simulink model "pv_trial"  (R2013a)
settings: Solver=ode4  StartTime=0.0  StopTime=0.2  FixedStep=1e-5  MaxStep=1e-5  RelTol=1e-3
values from neighbouring files (symbols this model uses):
  delta = atan(Idpv*Xs/(Vs-Iqpv*Xs))*180/pi    [rpg_simulation_base.m]
  fs = 50    [rpg_loss_calculation.m]    (also in rpg_simulation_base.m)
  fsw = 5e3    (= 5000)    [calculate_loss.m]    (also in rpg_loss_calculation.m; rpg_simulation_base.m = 2000)
  Ls = 1e-3    (= 0.001)    [rpg_simulation_base.m]
  ma = Vc_mag*sqrt(2)/Vdc    [rpg_simulation_base.m]
  Vdc = 750    [calculate_loss.m]    (also in rpg_loss_calculation.m; rpg_simulation_base.m)
  Vs = 400    [rpg_simulation_base.m]
libraries: powerlib x11, powerlib_extras x6, powerlib_meascontrol x4
settings Model: Creator=mesutto  LastModifiedBy=ugurm

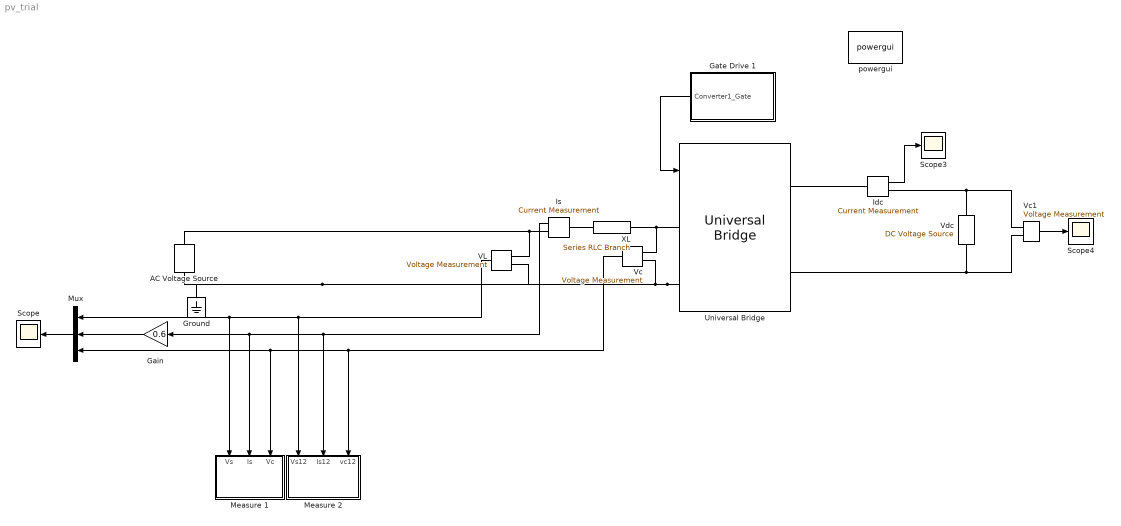
== system pv_trial ==
  AC Voltage Source : powerlib/Electrical Sources/AC Voltage Source  Amplitude=Vs*sqrt(2)  Phase=0  Frequency=50  SampleTime=0  Measurements=None
  Gain : Gain  Gain=0.6
  Gate Drive 1 : Subsystem
  Ground : powerlib/Elements/Ground  LConnTagsString=a
  Idc : powerlib/Measurements/Current Measurement  PhasorSimulation=off  OutputType=Complex  PSBequivalent=0
  Is : powerlib/Measurements/Current Measurement  PhasorSimulation=off  OutputType=Complex  PSBequivalent=0
  Measure 1 : Subsystem
  Measure 2 : Subsystem
  Mux : Mux  Inputs=3
  Scope : Scope
      settings: YMin=-3000  YMax=4500
  Scope3 : Scope
      settings: YMin=-2  YMax=2  SaveName=ScopeData3
  Scope4 : Scope
      settings: YMin=-2  YMax=2  SaveName=ScopeData4
  Universal Bridge : powerlib/Power Electronics/Universal Bridge  Arms=2  SnubberResistance=1e5  SnubberCapacitance=inf  Device=MOSFET / Diodes  Ron=1e-3  Lon=0  ForwardVoltages="[  0  0  ]"  ForwardVoltage=0  GTOparameters=[ 10e-6 , 20e-6 ]  IGBTparameters=[ 1e-6 , 2e-6 ]  Measurements=Device currents  Measurements_2=None  converterType=Rectifier
  VL : powerlib/Measurements/Voltage Measurement  PhasorSimulation=off  OutputType=Complex  PSBequivalent=0
  Vc : powerlib/Measurements/Voltage Measurement  PhasorSimulation=off  OutputType=Complex  PSBequivalent=0
  Vc1 : powerlib/Measurements/Voltage Measurement  PhasorSimulation=off  OutputType=Complex  PSBequivalent=0
  Vdc : powerlib/Electrical Sources/DC Voltage Source  Amplitude=Vdc  Measurements=None
  XL : powerlib/Elements/Series RLC Branch  LConnTagsString=__new0  RConnTagsString=__new0  BranchType=L  Resistance=1  Inductance=Ls  SetiL0=off  InitialCurrent=0  Capacitance=1e-6  Setx0=off  InitialVoltage=0  Measurements=None
  powergui : powerlib/powergui  Priority=1  SimulationMode=Discrete  SolverType=Tustin  SampleTime=1e-5  frequency=60  SPID=off  DisableSnubberDevices=off  DisableRonSwitches=off  DisableVfSwitches=off  SwTol=0  Interpol=off  DisplayEquations=off  frequencyindice=0  Pbase=100e6  ErrMax=1e-4  Iterations=50  UnitsV=kV  UnitsW=MW  FunctionMessages=off  echomessages=off  HookPort=off  EnableUseOfTLC=off  x0status=blocks  RestoreLinks=warning  ResistiveCurrentMeasurement=off  Frange=[0:2:500]  Ylog=off  Xlog=on  ShowGrid=off  save=off  variable=ZData  structure=h_vc  ZoomFFT=off  StartTime=0.02  cycles=5  DisplayStyle=1  fundamental=50  FreqAxis=off  MaxFrequency=4000  frequencyindicesteady=1  RmsSteady=1  display=off  Ts=0  methode=off
  wires:
  VL/1 -> Mux/1, Measure 1/1(Vs), Measure 2/1(Vs12)
  Mux/1 -> Scope/1
  Idc/1 -> Scope3/1
  Is/1 -> Gain/1, Measure 1/2(Is), Measure 2/2(Is12)
  Gain/1 -> Mux/2
  Vc/1 -> Mux/3, Measure 1/3(Vc), Measure 2/3(vc12)
  Vc1/1 -> Scope4/1
  Gate Drive 1/1(Converter1_Gate) -> Universal Bridge/1
  connections:
  XL/RConn1 -- Universal Bridge/LConn1 -- Vc/LConn1
  Idc/LConn1 -- Universal Bridge/RConn1
  Idc/RConn1 -- Vdc/RConn1 -- Vc1/LConn1
  Vc1/LConn2 -- Universal Bridge/RConn2 -- Vdc/LConn1
  AC Voltage Source/RConn1 -- Is/RConn1 -- VL/LConn1
  Universal Bridge/LConn2 -- AC Voltage Source/LConn1 -- Ground/LConn1 -- VL/LConn2 -- Vc/LConn2
  Is/LConn1 -- XL/LConn1

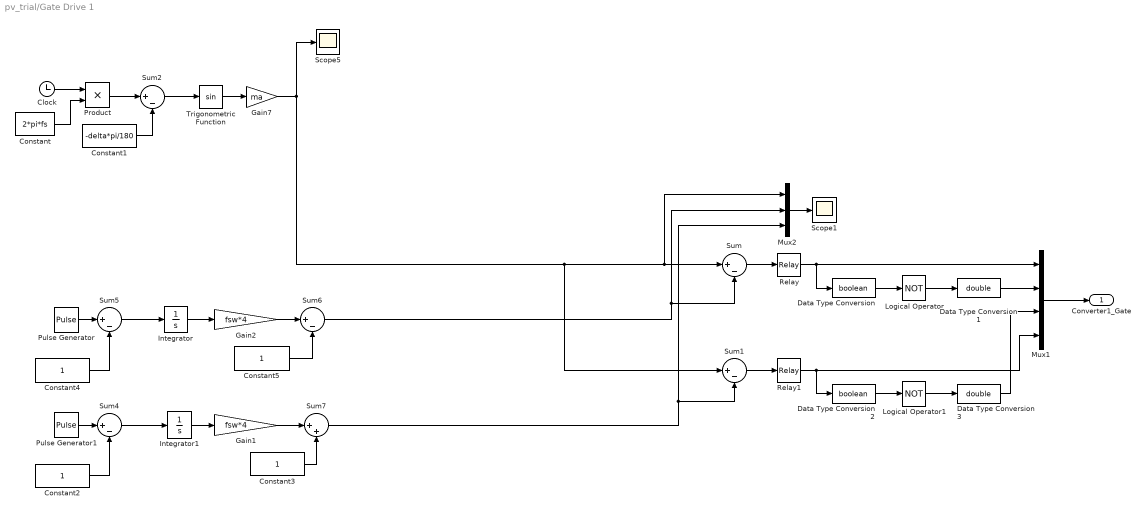
== system pv_trial/Gate Drive 1 ==
  Clock : Clock
  Constant : Constant  Value=2*pi*fs
  Constant1 : Constant  Value=-delta*pi/180
  Constant{2..5} (4 alike) : Constant
  Data Type Conversion : DataTypeConversion  OutDataTypeStr=boolean
  Data Type Conversion1 : DataTypeConversion  OutDataTypeStr=double
  Data Type Conversion2 : DataTypeConversion  OutDataTypeStr=boolean
  Data Type Conversion3 : DataTypeConversion  OutDataTypeStr=double
  Gain1 : Gain  Gain=fsw*4
  Gain2 : Gain  Gain=fsw*4
  Gain7 : Gain  Gain=ma
  Integrator : Integrator  ZeroCross=off
  Integrator1 : Integrator  ZeroCross=off
  Logical Operator : Logic  Operator=NOT  AllPortsSameDT=off  OutDataTypeStr=boolean
  Logical Operator1 : Logic  Operator=NOT  AllPortsSameDT=off  OutDataTypeStr=boolean
  Mux1 : Mux
  Mux2 : Mux  Inputs=3
  Product : Product
  Pulse Generator : DiscretePulseGenerator  PulseType=Time based  Amplitude=2  Period=1/fsw  PulseWidth=50
  Pulse Generator1 : DiscretePulseGenerator  PulseType=Time based  Amplitude=2  Period=1/fsw  PulseWidth=50  PhaseDelay=(1/fsw)/2
  Relay : Relay
  Relay1 : Relay
  Scope1 : Scope
      settings: YMin=-1.1  YMax=1.1
  Scope5 : Scope
      settings: YMin=-0.9  YMax=0.9  SaveName=ScopeData5
  Sum{,1..2,4..6} (6 alike) : Sum  Inputs=|+-
  Sum7 : Sum  Inputs=|++
  Trigonometric Function : Trigonometry
  Converter1_Gate : Outport
  wires:
  Relay1/1 -> Mux1/4, Data Type Conversion2/1
  Sum2/1 -> Trigonometric Function/1
  Trigonometric Function/1 -> Gain7/1
  Clock/1 -> Product/1
  Constant/1 -> Product/2
  Constant1/1 -> Sum2/2
  Product/1 -> Sum2/1
  Sum6/1 -> Mux2/2, Sum/2
  Sum/1 -> Relay/1
  Relay/1 -> Mux1/1, Data Type Conversion/1
  Data Type Conversion/1 -> Logical Operator/1
  Logical Operator/1 -> Data Type Conversion1/1
  Sum1/1 -> Relay1/1
  Data Type Conversion2/1 -> Logical Operator1/1
  Data Type Conversion1/1 -> Mux1/2
  Logical Operator1/1 -> Data Type Conversion3/1
  Mux1/1 -> Converter1_Gate/1
  Mux2/1 -> Scope1/1
  Gain7/1 -> Mux2/1, Sum/1, Sum1/1, Scope5/1
  Sum7/1 -> Sum1/2, Mux2/3
  Data Type Conversion3/1 -> Mux1/3
  Sum5/1 -> Integrator/1
  Integrator/1 -> Gain2/1
  Pulse Generator/1 -> Sum5/1
  Constant4/1 -> Sum5/2
  Gain2/1 -> Sum6/1
  Constant5/1 -> Sum6/2
  Sum4/1 -> Integrator1/1
  Integrator1/1 -> Gain1/1
  Pulse Generator1/1 -> Sum4/1
  Constant2/1 -> Sum4/2
  Gain1/1 -> Sum7/1
  Constant3/1 -> Sum7/2

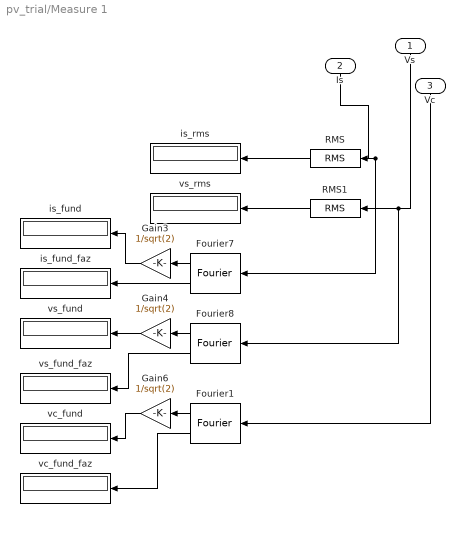
== system pv_trial/Measure 1 ==
  Vs : Inport
  Is : Inport  Port=2
  Vc : Inport  Port=3
  Fourier1 : powerlib_meascontrol/Measurements/Fourier  Freq=50  n=1  InInit=[0, 0]  Ts=0
  Fourier7 : powerlib_meascontrol/Measurements/Fourier  Freq=50  n=1  InInit=[0, 0]  Ts=0
  Fourier8 : powerlib_meascontrol/Measurements/Fourier  Freq=50  n=1  InInit=[0, 0]  Ts=0
  Gain3 : Gain  Gain=1/sqrt(2)
  Gain4 : Gain  Gain=1/sqrt(2)
  Gain6 : Gain  Gain=1/sqrt(2)
  RMS : powerlib_extras/Measurements/RMS  f1=50
  RMS1 : powerlib_extras/Measurements/RMS  f1=50
  is_fund : Display
  is_fund_faz : Display
  is_rms : Display
  vc_fund : Display
  vc_fund_faz : Display
  vs_fund : Display
  vs_fund_faz : Display
  vs_rms : Display
  wires:
  Vc/1 -> Fourier1/1
  Vs/1 -> Fourier8/1, RMS1/1
  Is/1 -> Fourier7/1, RMS/1
  Fourier7/2 -> is_fund_faz/1
  Fourier1/2 -> vc_fund_faz/1
  Fourier8/2 -> vs_fund_faz/1
  Gain3/1 -> is_fund/1
  Fourier1/1 -> Gain6/1
  Gain6/1 -> vc_fund/1
  Gain4/1 -> vs_fund/1
  RMS1/1 -> vs_rms/1
  RMS/1 -> is_rms/1
  Fourier7/1 -> Gain3/1
  Fourier8/1 -> Gain4/1

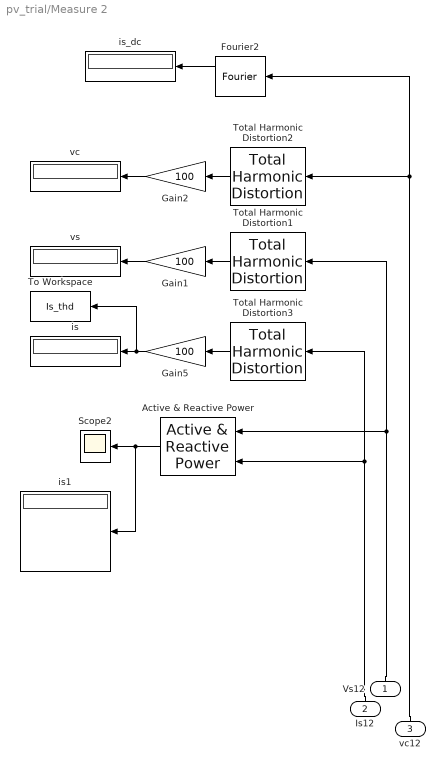
== system pv_trial/Measure 2 ==
  Vs12 : Inport
  Is12 : Inport  Port=2
  vc12 : Inport  Port=3
  Active & Reactive Power : powerlib_extras/Measurements/Active & Reactive Power  f1=50
  Fourier2 : powerlib_meascontrol/Measurements/Fourier  Freq=50  n=0  InInit=[0, 0]  Ts=0
  Gain1 : Gain  Gain=100
  Gain2 : Gain  Gain=100
  Gain5 : Gain  Gain=100
  Scope2 : Scope
      settings: YMin=-100  YMax=2000  SaveName=ScopeData2
  To Workspace : ToWorkspace  VariableName=Is_thd  SampleTime=1e-5  SaveFormat=Timeseries
  Total Harmonic Distortion1 : powerlib_extras/Measurements/Total Harmonic Distortion  f1=50
  Total Harmonic Distortion2 : powerlib_extras/Measurements/Total Harmonic Distortion  f1=50
  Total Harmonic Distortion3 : powerlib_extras/Measurements/Total Harmonic Distortion  f1=50
  is : Display
  is1 : Display
      settings: Format=bank
  is_dc : Display
  vc : Display
  vs : Display
  wires:
  Vs12/1 -> Active & Reactive Power/1, Total Harmonic Distortion1/1
  vc12/1 -> Fourier2/1, Total Harmonic Distortion2/1
  Is12/1 -> Active & Reactive Power/2, Total Harmonic Distortion3/1
  Fourier2/1 -> is_dc/1
  Gain5/1 -> To Workspace/1, is/1
  Total Harmonic Distortion3/1 -> Gain5/1
  Gain1/1 -> vs/1
  Total Harmonic Distortion1/1 -> Gain1/1
  Total Harmonic Distortion2/1 -> Gain2/1
  Gain2/1 -> vc/1
  Active & Reactive Power/1 -> is1/1, Scope2/1
